simulink model "RCAMAircraftSim"  (R2023b)
settings: Solver=VariableStepAuto  StartTime=0.0  StopTime=500  RelTol=1e-3
undefined symbols (not defined in the file or in its folder): RCAM_model, XStar
settings Model: Creator=shivashakeri  LastModifiedBy=shivashakeri

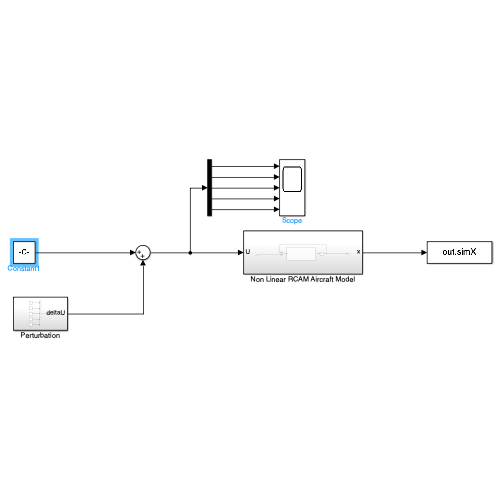
[thumbnail: Simulink's stored preview of the top-level diagram]
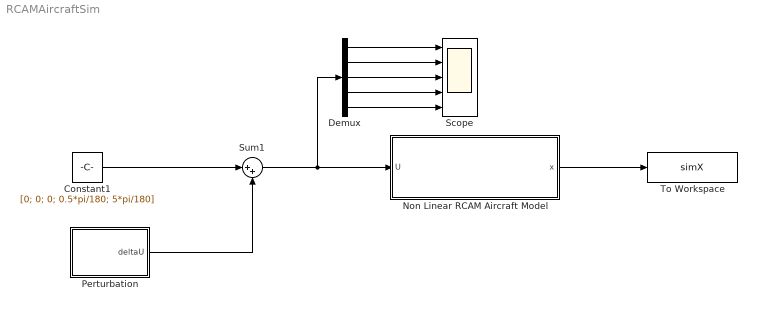
== system RCAMAircraftSim ==
  Constant1 : Constant  Value=[0; 0; 0; 0.5*pi/180; 5*pi/180]
  Demux : Demux  Outputs=5
  Non Linear RCAM Aircraft Model : Subsystem
  Perturbation : Subsystem
  Scope : Scope  NumInputPorts=5
  Sum1 : Sum  Inputs=|++
  To Workspace : ToWorkspace  VariableName=simX  SaveFormat=Timeseries  SampleTime=-1
  wires:
  Sum1/1 -> Demux/1, Non Linear RCAM Aircraft Model/1(U)
  Non Linear RCAM Aircraft Model/1(x) -> To Workspace/1
  Demux/1 -> Scope/1
  Demux/2 -> Scope/2
  Demux/3 -> Scope/3
  Demux/4 -> Scope/4
  Demux/5 -> Scope/5
  Perturbation/1(deltaU) -> Sum1/2
  Constant1/1 -> Sum1/1

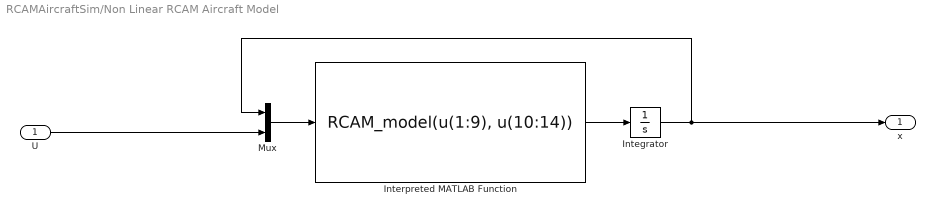
== system RCAMAircraftSim/Non Linear RCAM Aircraft Model ==
  U : Inport
  Integrator : Integrator  InitialCondition=XStar
  Interpreted MATLAB Function : MATLABFcn  MATLABFcn=RCAM_model(u(1:9), u(10:14))
  Mux : Mux  Inputs=2
  x : Outport
  wires:
  Interpreted MATLAB Function/1 -> Integrator/1
  Integrator/1 -> Mux/1, x/1
  U/1 -> Mux/2
  Mux/1 -> Interpreted MATLAB Function/1

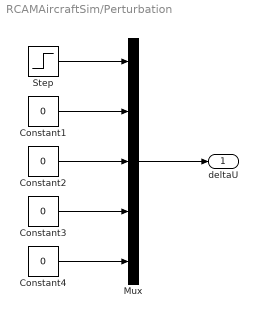
== system RCAMAircraftSim/Perturbation ==
  Constant{1..4} (4 alike) : Constant  Value=0
  Mux : Mux  Inputs=5
  Step : Step  After=0  SampleTime=0
  deltaU : Outport
  wires:
  Mux/1 -> deltaU/1
  Constant1/1 -> Mux/2
  Step/1 -> Mux/1
  Constant3/1 -> Mux/4
  Constant2/1 -> Mux/3
  Constant4/1 -> Mux/5
